simulink model "gm_tx80211a6l_interface"  (R2015b)
settings: Solver=FixedStepDiscrete  SolverMode=SingleTasking  StartTime=0.0  StopTime=46*tpf  RelTol=1e-3
PreLoadFcn:
  | [stx, stb, spi, spq, ntf, cii, cpp, css] = tx80211a_r0;
InitFcn:
  | if ~exist('srx','var')
  | [stx, stb, spi, spq, ntf, cii, cpp, css] = tx80211a_r0;
  | end
  | bitrate = 6e6; % 6 Mbits per second
  | crf = 2; % constant redundancy factor (from conv enc)
  | nepsc = 16; % #empty+pilot subcarriers
  | ncps = 16; % #cyclic prefix samples
  | ndbpf = 24; % #data bits per frame
  | ncbpf = ndbpf * crf; % #coded bits per frame
  | nscpf = ncbpf + nepsc; % #subcarriers per frame
  | nspf = nscpf + 16; % #samples per frame
  | tps = 1e-6; %tpf/nspf; % sample time
  | tpf = tps*nspf; %ndbpf/bitrate; % frame time
undefined symbols (not defined in the file): AXI4, css, Lite, ntf, stb
libraries: hdlsllib x30, simulink x13, axiinterfacelib x4, dspsigops x2
settings Model: SimulationMode=external  Creator=wchen  LastModifiedBy=bdroz
settings SolverCC: PositivePriorityOrder=on
settings DataIOCC: SaveFormat=Array  SaveOutput=off  SignalLogging=off  SaveTime=off
settings OptimizationCC: BlockReduction=off  ConditionallyExecuteInputs=off  ExpressionDepthLimit=2147483647  OptimizeModelRefInitCode=on  LifeSpan=1  MaxStackSize=64
settings DebuggingCC: AlgebraicLoopMsg=error  UnderspecifiedInitializationDetection=Classic  MergeDetectMultiDrivingBlocksExec=none  SolverPrmCheckMsg=warning  SingleTaskRateTransMsg=error  ParameterPrecisionLossMsg=none  AllowSymbolicDim=on  StateNameClashWarn=warning
settings HardwareCC: ProdBitPerPointer=32  ProdLargestAtomicInteger=Long  ProdLargestAtomicFloat=Double  ProdWordSize=32  ProdHWDeviceType=ARM Compatible->ARM Cortex  TargetBitPerPointer=64  TargetLongLongMode=on  TargetIntDivRoundTo=Zero  TargetEndianess=LittleEndian  TargetWordSize=64  TargetHWDeviceType=MATLAB Host
settings RTWCC: SystemTargetFile=ert.tlc  TemplateMakefile=ert_default_tmf  Description=Embedded Coder  GenerateReport=on  Toolchain=Xilinx Software Development Kit (SDK)  IncludeHyperlinkInReport=on  LaunchReport=on  GenerateTraceInfo=on  GenerateTraceReport=on  GenerateTraceReportSl=on  GenerateTraceReportSf=on  GenerateTraceReportEml=on
settings CodeAppCC: ForceParamTrailComments=on  IgnoreCustomStorageClasses=off  OperatorAnnotations=on  SimulinkDataObjDesc=on  SFDataObjDesc=on  MATLABFcnDesc=on  InsertBlockDesc=on  MATLABSourceComments=on
settings ERTTargetCC: ConvertIfToSwitch=on  SuppressUnreachableDefaultCases=on
settings ConfigComp: CovModelRefEnable=Off

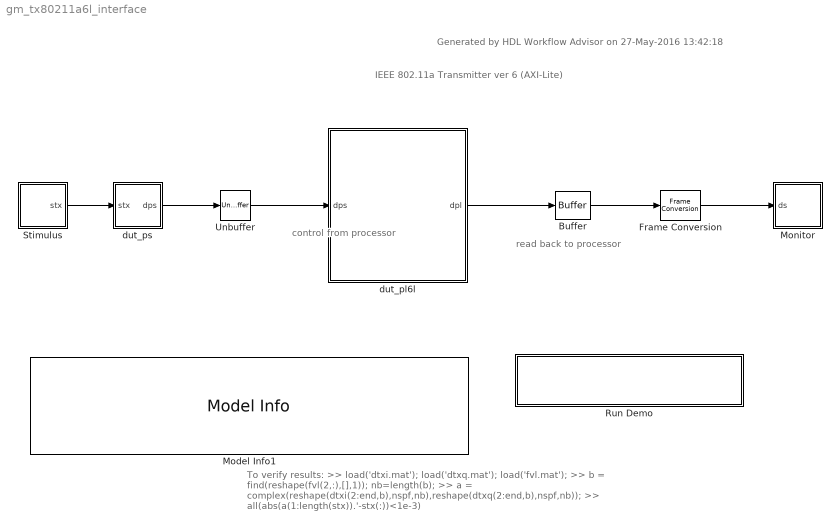
== system gm_tx80211a6l_interface ==
  note: To verify results:
      | >> load('dtxi.mat'); load('dtxq.mat'); load('fvl.mat');
      | >> b = find(reshape(fvl(2,:),[],1)); nb=length(b);
      | >> a = complex(reshape(dtxi(2:end,b),nspf,nb),reshape(dtxq(2:end,b),nspf,nb));
      | >> all(abs(a(1:length(stx)).'-stx(:))<1e-3)
  note: read back to
      | processor
  note: IEEE 802.11a Transmitter ver 6 (AXI-Lite)
  note: control from
      | processor
  note: Generated by HDL Workflow Advisor on 27-May-2016 13:42:18
  Buffer : Buffer  N=nspf  TreatMby1Signals=One channel  OutputFrames=off
  Frame Conversion : FrameConversion  InheritSamplingMode=off  OutFrame=Sample-based
  Model Info1 : simulink/Model-Wide Utilities/Model Info  Frame=on  DisplayStringWithTags=|  HorizontalTextAlignment=Left  LeftAlignmentValue=0.02  SourceBlockDiagram=gm_tx80211a6l_interface  TagMaxNumber=20
      | This example shows how to use HDL Workflow Advisor to 
      | generate a custom IP core for Zynq SoC evaluation board.
      | 
      | In MATLAB, type the following:
      |   hdladvisor('tx80211a6l/dut_pl6l')
  Monitor : Subsystem
  Run Demo : Subsystem
      settings: OpenFcn=hdladvisor([bdroot, '/led_counter'])
      mask Display: disp('Launch HDL Workflow Advisor')
  Stimulus : Subsystem
  Unbuffer : Unbuffer  SampleBasedProcessing=Same as frame based
  dut_pl6l : Subsystem  TreatAsAtomicUnit=on  mask(AXI4-Lite/AXI4 Interface){}
      mask help:
      | This is an automatically generated subsystem block.
      | This contains the AXI interface blocks that communicate with the tx80211a6l_dut_pl6l_ipcore IPCore generated from tx80211a6l/dut_pl6l subsystem.
      mask Display: disp(sprintf('Xilinx Zynq \nAXI Interface'));
  dut_ps : Subsystem
  wires:
  Frame Conversion/1 -> Monitor/1(ds)
  Unbuffer/1 -> dut_pl6l/1(dps)
  dut_ps/1(dps) -> Unbuffer/1
  Stimulus/1(stx) -> dut_ps/1(stx)
  dut_pl6l/1(dpl) -> Buffer/1
  Buffer/1 -> Frame Conversion/1

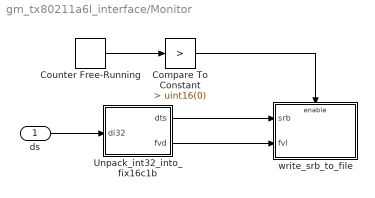
== system gm_tx80211a6l_interface/Monitor ==
  ds : Inport
  Compare To Constant : simulink/Logic and Bit Operations/Compare To Constant  relop=>  const=uint16(0)  OutDataTypeStr=boolean
  Counter Free-Running : simulink/Sources/Counter Free-Running  NumBits=16  tsamp=tpf
  Unpack_int32_into_fix16c1b : Subsystem
  write_srb_to_file : Subsystem
  wires:
  Unpack_int32_into_fix16c1b/1(dts) -> write_srb_to_file/1(srb)
  Unpack_int32_into_fix16c1b/2(fvd) -> write_srb_to_file/2(fvl)
  ds/1 -> Unpack_int32_into_fix16c1b/1(di32)
  Counter Free-Running/1 -> Compare To Constant/1
  Compare To Constant/1 -> write_srb_to_file/Enable

== system gm_tx80211a6l_interface/Run Demo ==

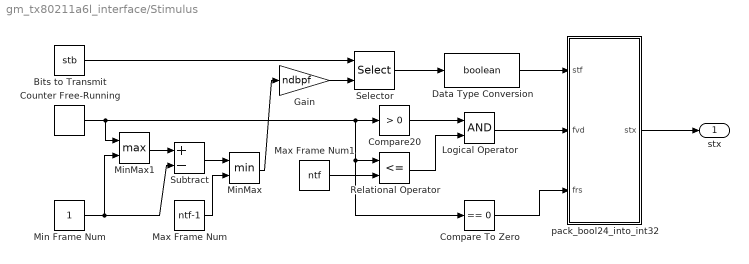
== system gm_tx80211a6l_interface/Stimulus ==
  Bits to Transmit : Constant  Value=stb  SampleTime=tpf
  Compare To Zero : simulink/Logic and Bit Operations/Compare To Zero  relop===  OutDataTypeStr=boolean
  Compare20 : simulink/Logic and Bit Operations/Compare To Zero  relop=>  OutDataTypeStr=boolean
  Counter Free-Running : simulink/Sources/Counter Free-Running  NumBits=16  tsamp=tpf
  Data Type Conversion : DataTypeConversion  OutDataTypeStr=boolean
  Gain : Gain  Gain=ndbpf  OutDataTypeStr=uint16
  Logical Operator : Logic  AllPortsSameDT=off  OutDataTypeStr=boolean
  Max Frame Num : Constant  Value=ntf-1  OutDataTypeStr=uint16  SampleTime=tpf
  Max Frame Num1 : Constant  Value=ntf  OutDataTypeStr=uint16  SampleTime=tpf
  Min Frame Num : Constant  OutDataTypeStr=uint16  SampleTime=tpf
  MinMax : MinMax  Inputs=2  OutDataTypeStr=uint16
  MinMax1 : MinMax  Function=max  Inputs=2
  Relational Operator : RelationalOperator  Operator=<=  OutDataTypeStr=boolean
  Selector : Selector  IndexMode=Zero-based  InputPortWidth=864  IndexOptions=Starting index (port)  Indices=[1 3]  OutputSizes=24
  Subtract : Sum  Inputs=+-  OutDataTypeStr=uint16
  pack_bool24_into_int32 : Subsystem
  stx : Outport
  wires:
  Max Frame Num1/1 -> Relational Operator/2
  Logical Operator/1 -> pack_bool24_into_int32/2(fvd)
  Relational Operator/1 -> Logical Operator/2
  Compare20/1 -> Logical Operator/1
  Counter Free-Running/1 -> MinMax1/1, Compare To Zero/1, Relational Operator/1, Compare20/1
  Max Frame Num/1 -> MinMax/2
  MinMax/1 -> Gain/1
  Bits to Transmit/1 -> Selector/1
  Gain/1 -> Selector/2
  Selector/1 -> Data Type Conversion/1
  Data Type Conversion/1 -> pack_bool24_into_int32/1(stf)
  pack_bool24_into_int32/1(stx) -> stx/1
  Min Frame Num/1 -> Subtract/2, MinMax1/2
  Subtract/1 -> MinMax/1
  MinMax1/1 -> Subtract/1
  Compare To Zero/1 -> pack_bool24_into_int32/3(frs)

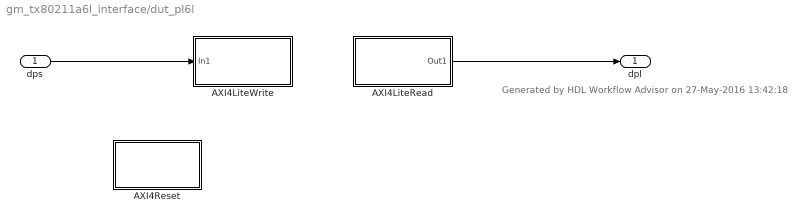
== system gm_tx80211a6l_interface/dut_pl6l ==
  note: Generated by HDL Workflow Advisor on 27-May-2016 13:42:18
  dps : Inport
  AXI4LiteRead : Subsystem  Priority=10
  AXI4LiteWrite : Subsystem  Priority=1
  AXI4Reset : Subsystem  mask(System Initialize){ShowInLibBrowser=0}
      mask prompts: ShowInLibBrowser "Simulink:masks:CustCodeMaskParam1_MP"
      settings: CopyFcn=cccopyfcn(gcb)  OpenFcn=ccopenfcn('System Initialize Function')
      mask Help: eval('feval(''rtwprivate'',''rtwhelpview'',''rtw_sys_initialize_block'')');
      mask Display: disp('System\nInitialize');
  dpl : Outport  InitialOutput=0
  wires:
  dps/1 -> AXI4LiteWrite/1(In1)
  AXI4LiteRead/1(Out1) -> dpl/1

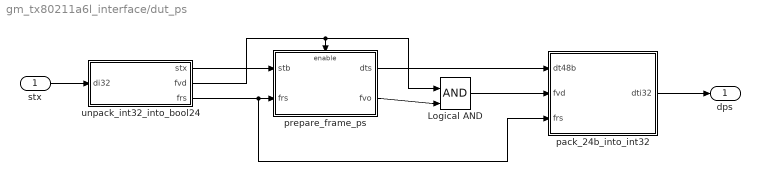
== system gm_tx80211a6l_interface/dut_ps ==
  stx : Inport
  Logical AND : Logic  IconShape=distinctive  AllPortsSameDT=off  OutDataTypeStr=boolean
  pack_24b_into_int32 : Subsystem
  prepare_frame_ps : Subsystem  TreatAsAtomicUnit=on
  unpack_int32_into_bool24 : Subsystem
  dps : Outport
  wires:
  prepare_frame_ps/2(fvo) -> Logical AND/2
  Logical AND/1 -> pack_24b_into_int32/2(fvd)
  pack_24b_into_int32/1(dti32) -> dps/1
  prepare_frame_ps/1(dts) -> pack_24b_into_int32/1(dt48b)
  unpack_int32_into_bool24/2(fvd) -> prepare_frame_ps/Enable, Logical AND/1
  unpack_int32_into_bool24/1(stx) -> prepare_frame_ps/1(stb)
  unpack_int32_into_bool24/3(frs) -> prepare_frame_ps/2(frs), pack_24b_into_int32/3(frs)
  stx/1 -> unpack_int32_into_bool24/1(di32)

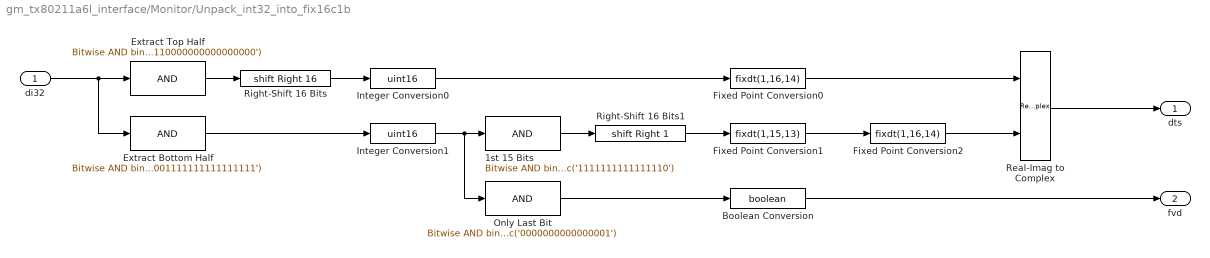
== system gm_tx80211a6l_interface/Monitor/Unpack_int32_into_fix16c1b ==
  di32 : Inport
  1st 15 Bits : simulink/Logic and Bit Operations/Bitwise Operator  logicop=AND  UseBitMask=on  BitMask=bin2dec('1111111111111110')  BitMaskRealWorld=Stored Integer
  Boolean Conversion : DataTypeConversion  OutDataTypeStr=boolean  ConvertRealWorld=Stored Integer (SI)
  Extract Bottom Half : simulink/Logic and Bit Operations/Bitwise Operator  logicop=AND  UseBitMask=on  BitMask=bin2dec('00000000000000001111111111111111')  BitMaskRealWorld=Stored Integer
  Extract Top Half : simulink/Logic and Bit Operations/Bitwise Operator  logicop=AND  UseBitMask=on  BitMask=bin2dec('11111111111111110000000000000000')  BitMaskRealWorld=Stored Integer
  Fixed Point Conversion0 : DataTypeConversion  OutDataTypeStr=fixdt(1,16,14)  ConvertRealWorld=Stored Integer (SI)
      settings: AttributesFormatString=%<OutDataTypeStr>
  Fixed Point Conversion1 : DataTypeConversion  OutDataTypeStr=fixdt(1,15,13)  ConvertRealWorld=Stored Integer (SI)
      settings: AttributesFormatString=%<OutDataTypeStr>
  Fixed Point Conversion2 : DataTypeConversion  OutDataTypeStr=fixdt(1,16,14)
      settings: AttributesFormatString=%<OutDataTypeStr>
  Integer Conversion0 : DataTypeConversion  OutDataTypeStr=uint16  ConvertRealWorld=Stored Integer (SI)
  Integer Conversion1 : DataTypeConversion  OutDataTypeStr=uint16  ConvertRealWorld=Stored Integer (SI)
  Only Last Bit : simulink/Logic and Bit Operations/Bitwise Operator  logicop=AND  UseBitMask=on  BitMask=bin2dec('0000000000000001')  BitMaskRealWorld=Stored Integer
  Real-Imag to Complex : RealImagToComplex
  Right-Shift 16 Bits : ArithShift  BitShiftNumber=16  BitShiftDirection=Right  DiagnosticForOORShift=Error
  Right-Shift 16 Bits1 : ArithShift  BitShiftNumber=1  BitShiftDirection=Right  DiagnosticForOORShift=Error
  dts : Outport
  fvd : Outport  Port=2
  wires:
  Right-Shift 16 Bits1/1 -> Fixed Point Conversion1/1
  Fixed Point Conversion1/1 -> Fixed Point Conversion2/1
  Integer Conversion0/1 -> Fixed Point Conversion0/1
  Integer Conversion1/1 -> Only Last Bit/1, 1st 15 Bits/1
  Extract Top Half/1 -> Right-Shift 16 Bits/1
  Right-Shift 16 Bits/1 -> Integer Conversion0/1
  1st 15 Bits/1 -> Right-Shift 16 Bits1/1
  di32/1 -> Extract Top Half/1, Extract Bottom Half/1
  Extract Bottom Half/1 -> Integer Conversion1/1
  Fixed Point Conversion2/1 -> Real-Imag to Complex/2
  Fixed Point Conversion0/1 -> Real-Imag to Complex/1
  Boolean Conversion/1 -> fvd/1
  Only Last Bit/1 -> Boolean Conversion/1
  Real-Imag to Complex/1 -> dts/1

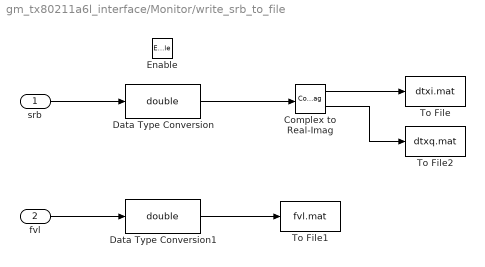
== system gm_tx80211a6l_interface/Monitor/write_srb_to_file ==
  srb : Inport
  fvl : Inport  Port=2
  Enable : EnablePort
  Complex to Real-Imag : ComplexToRealImag
  Data Type Conversion : DataTypeConversion  OutDataTypeStr=double
  Data Type Conversion1 : DataTypeConversion  OutDataTypeStr=double
  To File : ToFile  Filename=dtxi.mat  MatrixName=dtxi  SampleTime=tpf
  To File1 : ToFile  Filename=fvl.mat  MatrixName=fvl  SampleTime=tpf
  To File2 : ToFile  Filename=dtxq.mat  MatrixName=dtxq  SampleTime=tpf
  wires:
  Complex to Real-Imag/2 -> To File2/1
  Complex to Real-Imag/1 -> To File/1
  Data Type Conversion/1 -> Complex to Real-Imag/1
  srb/1 -> Data Type Conversion/1
  Data Type Conversion1/1 -> To File1/1
  fvl/1 -> Data Type Conversion1/1

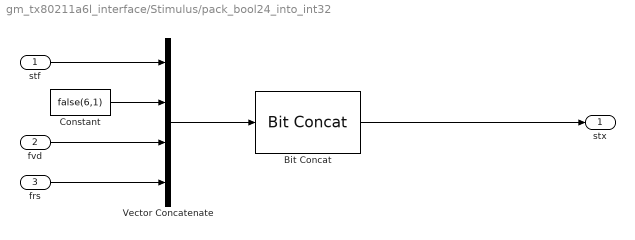
== system gm_tx80211a6l_interface/Stimulus/pack_bool24_into_int32 ==
  stf : Inport
  fvd : Inport  Port=2
  frs : Inport  Port=3
  Bit Concat : hdlsllib/HDL Operations/Bit Concat  numInputs=1
  Constant : Constant  Value=false(6,1)  OutDataTypeStr=boolean  SampleTime=tpf
  Vector Concatenate : Concatenate  NumInputs=4
  stx : Outport
  wires:
  Bit Concat/1 -> stx/1
  Constant/1 -> Vector Concatenate/2
  frs/1 -> Vector Concatenate/4
  fvd/1 -> Vector Concatenate/3
  stf/1 -> Vector Concatenate/1
  Vector Concatenate/1 -> Bit Concat/1

== system gm_tx80211a6l_interface/dut_pl6l/AXI4LiteRead ==
  AXI4Lite_Read_dpl : axiinterfacelib/AXI4-Interface Read  Priority=2  AXIInterfaceType=AXI4-Lite  DeviceName=/dev/mwipcore  RegisterOffset=hex2dec('104')  DataLength=4096  DataType=uint32  SampleTime=-1  blockPlatform=ZYNQ  SimulateUsing=Interpreted Execution
  AXI4Lite_Read_dpl_DTC : DataTypeConversion  OutDataTypeStr=fixdt('uint32')  ConvertRealWorld=Stored Integer (SI)
  AXI4_Handshake : Subsystem  Priority=1  mask(AXI4-Lite/AXI4 Handshake){blockPlatform=ZYNQ}
      mask prompts: blockPlatform "Mask Parameter 1:"
      mask help:
      | This is an automatically generated block.
      | It synchronizes the data between ARM and FPGA on AXI4-Lite/AXI4 interface.
      |
      | This block writes the FPGA Strobe signal to indicate that the data from ARM on AXI4-Lite/AXI4 interface is valid.
      |
      | It waits until the FPGA Ready signal is 1 (logic-HIGH), which shows that data from FPGA on AXI4-Lite/AXI4 interface is valid.
      mask Display:
      | color('blue');
      | text(0.67, 0.87, 'ZYNQ', 'horizontalAlignment', 'left');
  Out1 : Outport
  wires:
  AXI4Lite_Read_dpl_DTC/1 -> Out1/1
  AXI4Lite_Read_dpl/1 -> AXI4Lite_Read_dpl_DTC/1

== system gm_tx80211a6l_interface/dut_pl6l/AXI4LiteWrite ==
  In1 : Inport
  AXI4Lite_Write_dps : axiinterfacelib/AXI4-Interface Write  Priority=1  AXIInterfaceType=AXI4-Lite  DeviceName=/dev/mwipcore  RegisterOffset=hex2dec('100')  blockPlatform=ZYNQ  SimulateUsing=Interpreted execution
  AXI4Lite_Write_dps_DTC : DataTypeConversion  OutDataTypeStr=uint32  ConvertRealWorld=Stored Integer (SI)
  wires:
  AXI4Lite_Write_dps_DTC/1 -> AXI4Lite_Write_dps/1
  In1/1 -> AXI4Lite_Write_dps_DTC/1

== system gm_tx80211a6l_interface/dut_pl6l/AXI4Reset ==

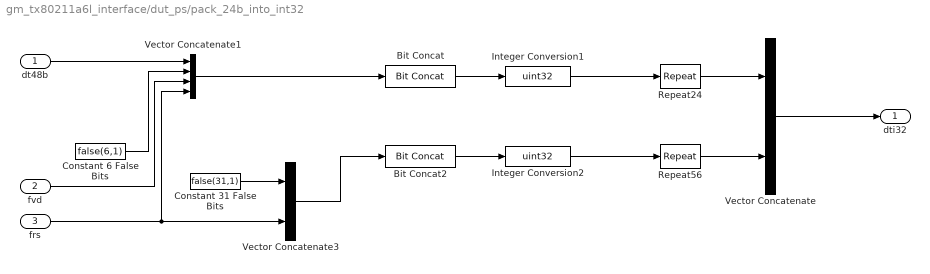
== system gm_tx80211a6l_interface/dut_ps/pack_24b_into_int32 ==
  dt48b : Inport
  fvd : Inport  Port=2
  frs : Inport  Port=3
  Bit Concat : hdlsllib/HDL Operations/Bit Concat  numInputs=1
  Bit Concat2 : hdlsllib/HDL Operations/Bit Concat  numInputs=1
  Constant 31 False Bits : Constant  Value=false(31,1)  OutDataTypeStr=boolean  SampleTime=tpf
  Constant 6 False Bits : Constant  Value=false(6,1)  OutDataTypeStr=boolean  SampleTime=tpf
  Integer Conversion1 : DataTypeConversion  OutDataTypeStr=uint32  ConvertRealWorld=Stored Integer (SI)
  Integer Conversion2 : DataTypeConversion  OutDataTypeStr=uint32  ConvertRealWorld=Stored Integer (SI)
  Repeat24 : dspsigops/Repeat  N=24  InputProcessing=Columns as channels (frame based)  RateOptions=Enforce single-rate processing  ic=0  mode=Unused parameter value
  Repeat56 : dspsigops/Repeat  N=56  InputProcessing=Columns as channels (frame based)  RateOptions=Enforce single-rate processing  ic=0  mode=Unused parameter value
  Vector Concatenate : Concatenate
  Vector Concatenate1 : Concatenate  NumInputs=4
  Vector Concatenate3 : Concatenate
  dti32 : Outport
  wires:
  Repeat24/1 -> Vector Concatenate/1
  Integer Conversion1/1 -> Repeat24/1
  Repeat56/1 -> Vector Concatenate/2
  Integer Conversion2/1 -> Repeat56/1
  Bit Concat2/1 -> Integer Conversion2/1
  Vector Concatenate3/1 -> Bit Concat2/1
  Constant 31 False Bits/1 -> Vector Concatenate3/1
  Constant 6 False Bits/1 -> Vector Concatenate1/2
  Vector Concatenate1/1 -> Bit Concat/1
  frs/1 -> Vector Concatenate3/2, Vector Concatenate1/4
  fvd/1 -> Vector Concatenate1/3
  dt48b/1 -> Vector Concatenate1/1
  Bit Concat/1 -> Integer Conversion1/1
  Vector Concatenate/1 -> dti32/1

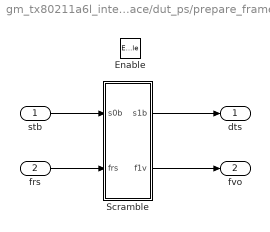
== system gm_tx80211a6l_interface/dut_ps/prepare_frame_ps ==
  stb : Inport
  frs : Inport  Port=2
  Enable : EnablePort
  Scramble : Subsystem  TreatAsAtomicUnit=on
  dts : Outport
  fvo : Outport  Port=2  InitialOutput=0
  wires:
  Scramble/1(s1b) -> dts/1
  Scramble/2(f1v) -> fvo/1
  frs/1 -> Scramble/2(frs)
  stb/1 -> Scramble/1(s0b)

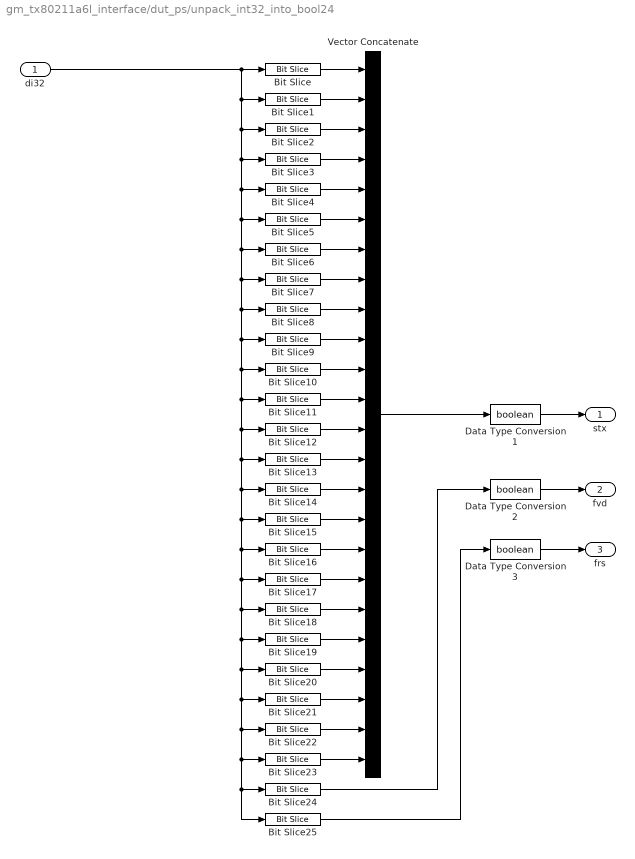
== system gm_tx80211a6l_interface/dut_ps/unpack_int32_into_bool24 ==
  di32 : Inport
  Bit Slice : hdlsllib/HDL Operations/Bit Slice  lidx=31  ridx=31
      settings: AttributesFormatString=%<lidx>
  Bit Slice1 : hdlsllib/HDL Operations/Bit Slice  lidx=30  ridx=30
      settings: AttributesFormatString=%<lidx>
  Bit Slice10 : hdlsllib/HDL Operations/Bit Slice  lidx=21  ridx=21
      settings: AttributesFormatString=%<lidx>
  Bit Slice11 : hdlsllib/HDL Operations/Bit Slice  lidx=20  ridx=20
      settings: AttributesFormatString=%<lidx>
  Bit Slice12 : hdlsllib/HDL Operations/Bit Slice  lidx=19  ridx=19
      settings: AttributesFormatString=%<lidx>
  Bit Slice13 : hdlsllib/HDL Operations/Bit Slice  lidx=18  ridx=18
      settings: AttributesFormatString=%<lidx>
  Bit Slice14 : hdlsllib/HDL Operations/Bit Slice  lidx=17  ridx=17
      settings: AttributesFormatString=%<lidx>
  Bit Slice15 : hdlsllib/HDL Operations/Bit Slice  lidx=16  ridx=16
      settings: AttributesFormatString=%<lidx>
  Bit Slice16 : hdlsllib/HDL Operations/Bit Slice  lidx=15  ridx=15
      settings: AttributesFormatString=%<lidx>
  Bit Slice17 : hdlsllib/HDL Operations/Bit Slice  lidx=14  ridx=14
      settings: AttributesFormatString=%<lidx>
  Bit Slice18 : hdlsllib/HDL Operations/Bit Slice  lidx=13  ridx=13
      settings: AttributesFormatString=%<lidx>
  Bit Slice19 : hdlsllib/HDL Operations/Bit Slice  lidx=12  ridx=12
      settings: AttributesFormatString=%<lidx>
  Bit Slice2 : hdlsllib/HDL Operations/Bit Slice  lidx=29  ridx=29
      settings: AttributesFormatString=%<lidx>
  Bit Slice20 : hdlsllib/HDL Operations/Bit Slice  lidx=11  ridx=11
      settings: AttributesFormatString=%<lidx>
  Bit Slice21 : hdlsllib/HDL Operations/Bit Slice  lidx=10  ridx=10
      settings: AttributesFormatString=%<lidx>
  Bit Slice22 : hdlsllib/HDL Operations/Bit Slice  lidx=9  ridx=9
      settings: AttributesFormatString=%<lidx>
  Bit Slice23 : hdlsllib/HDL Operations/Bit Slice  lidx=8  ridx=8
      settings: AttributesFormatString=%<lidx>
  Bit Slice24 : hdlsllib/HDL Operations/Bit Slice  lidx=1  ridx=1
      settings: AttributesFormatString=%<lidx>
  Bit Slice25 : hdlsllib/HDL Operations/Bit Slice  lidx=0  ridx=0
      settings: AttributesFormatString=%<lidx>
  Bit Slice3 : hdlsllib/HDL Operations/Bit Slice  lidx=28  ridx=28
      settings: AttributesFormatString=%<lidx>
  Bit Slice4 : hdlsllib/HDL Operations/Bit Slice  lidx=27  ridx=27
      settings: AttributesFormatString=%<lidx>
  Bit Slice5 : hdlsllib/HDL Operations/Bit Slice  lidx=26  ridx=26
      settings: AttributesFormatString=%<lidx>
  Bit Slice6 : hdlsllib/HDL Operations/Bit Slice  lidx=25  ridx=25
      settings: AttributesFormatString=%<lidx>
  Bit Slice7 : hdlsllib/HDL Operations/Bit Slice  lidx=24  ridx=24
      settings: AttributesFormatString=%<lidx>
  Bit Slice8 : hdlsllib/HDL Operations/Bit Slice  lidx=23  ridx=23
      settings: AttributesFormatString=%<lidx>
  Bit Slice9 : hdlsllib/HDL Operations/Bit Slice  lidx=22  ridx=22
      settings: AttributesFormatString=%<lidx>
  Data Type Conversion1 : DataTypeConversion  OutDataTypeStr=boolean
  Data Type Conversion2 : DataTypeConversion  OutDataTypeStr=boolean
  Data Type Conversion3 : DataTypeConversion  OutDataTypeStr=boolean
  Vector Concatenate : Concatenate  NumInputs=24
  stx : Outport
  fvd : Outport  Port=2
  frs : Outport  Port=3
  wires:
  Data Type Conversion3/1 -> frs/1
  Data Type Conversion2/1 -> fvd/1
  Data Type Conversion1/1 -> stx/1
  Bit Slice/1 -> Vector Concatenate/1
  Bit Slice1/1 -> Vector Concatenate/2
  Bit Slice2/1 -> Vector Concatenate/3
  Bit Slice3/1 -> Vector Concatenate/4
  Bit Slice4/1 -> Vector Concatenate/5
  Bit Slice5/1 -> Vector Concatenate/6
  Bit Slice6/1 -> Vector Concatenate/7
  Bit Slice7/1 -> Vector Concatenate/8
  Bit Slice8/1 -> Vector Concatenate/9
  Bit Slice9/1 -> Vector Concatenate/10
  Bit Slice10/1 -> Vector Concatenate/11
  Bit Slice11/1 -> Vector Concatenate/12
  Bit Slice12/1 -> Vector Concatenate/13
  Bit Slice13/1 -> Vector Concatenate/14
  Bit Slice14/1 -> Vector Concatenate/15
  Bit Slice15/1 -> Vector Concatenate/16
  Bit Slice16/1 -> Vector Concatenate/17
  Bit Slice17/1 -> Vector Concatenate/18
  Bit Slice18/1 -> Vector Concatenate/19
  Bit Slice19/1 -> Vector Concatenate/20
  Bit Slice20/1 -> Vector Concatenate/21
  Bit Slice21/1 -> Vector Concatenate/22
  Bit Slice22/1 -> Vector Concatenate/23
  Bit Slice23/1 -> Vector Concatenate/24
  di32/1 -> Bit Slice/1, Bit Slice6/1, Bit Slice10/1, Bit Slice14/1, Bit Slice16/1, Bit Slice22/1, Bit Slice23/1, Bit Slice24/1, Bit Slice25/1, Bit Slice21/1, Bit Slice20/1, Bit Slice19/1, Bit Slice18/1, Bit Slice17/1, Bit Slice15/1, Bit Slice13/1, Bit Slice12/1, Bit Slice11/1, Bit Slice9/1, Bit Slice8/1, Bit Slice7/1, Bit Slice5/1, Bit Slice4/1, Bit Slice3/1, Bit Slice2/1, Bit Slice1/1
  Bit Slice24/1 -> Data Type Conversion2/1
  Bit Slice25/1 -> Data Type Conversion3/1
  Vector Concatenate/1 -> Data Type Conversion1/1

== system gm_tx80211a6l_interface/dut_pl6l/AXI4LiteRead/AXI4_Handshake ==
  AXI4_Write_FPGA_STROBE : axiinterfacelib/AXI4-Interface Write  Priority=1  AXIInterfaceType=AXI4-Lite  DeviceName=/dev/mwipcore  RegisterOffset=hex2dec('8')  blockPlatform=ZYNQ  SimulateUsing=Interpreted execution
  Constant : Constant  OutDataTypeStr=uint32
  WhileIteratorSubsystem : Subsystem  Priority=10  TreatAsAtomicUnit=on
  wires:
  Constant/1 -> AXI4_Write_FPGA_STROBE/1

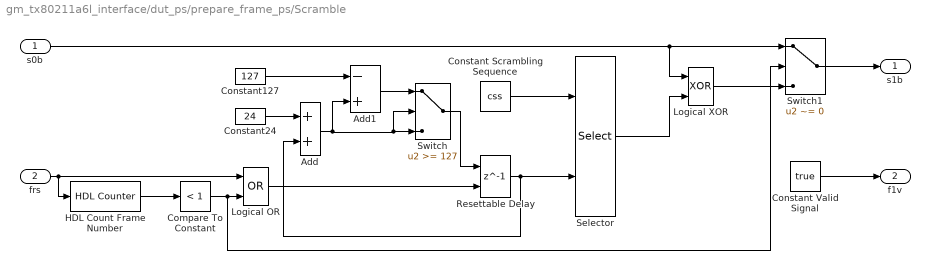
== system gm_tx80211a6l_interface/dut_ps/prepare_frame_ps/Scramble ==
  s0b : Inport
  frs : Inport  Port=2
  Add : Sum  AccumDataTypeStr=int16  OutDataTypeStr=int16  SaturateOnIntegerOverflow=on
  Add1 : Sum  Inputs=-+  AccumDataTypeStr=int16  OutDataTypeStr=int16  SaturateOnIntegerOverflow=on  LockScale=on
  Compare To Constant : simulink/Logic and Bit Operations/Compare To Constant  relop=<  const=1  OutDataTypeStr=boolean
  Constant Scrambling Sequence : Constant  Value=css  OutDataTypeStr=boolean  SampleTime=tpf
  Constant Valid Signal : Constant  Value=true  OutDataTypeStr=boolean  SampleTime=tpf
  Constant127 : Constant  Value=127  OutDataTypeStr=int16  SampleTime=tpf
  Constant24 : Constant  Value=24  OutDataTypeStr=int16  SampleTime=tpf
  HDL Count Frame Number : hdlsllib/HDL Operations/HDL Counter  CountType=Free running  CountInit=0  CountStep=1  CountMax=25  CountFromType=Initial value  CountFrom=0  CountResetPort=on  CountLoadPort=off  CountEnbPort=off  CountDirPort=off  CountDataType=Unsigned  CountWordLen=16  CountFracLen=0  CountSampTime=1
  Logical OR : Logic  Operator=OR  IconShape=distinctive  AllPortsSameDT=off  OutDataTypeStr=boolean
  Logical XOR : Logic  Operator=XOR  IconShape=distinctive  AllPortsSameDT=off  OutDataTypeStr=boolean
  Resettable Delay : Delay  DelayLength=1  InitialCondition=int16(0)  ExternalReset=Level  SampleTime=tpf
      settings: InputPortMap=u0,r5
  Selector : Selector  IndexMode=Zero-based  InputPortWidth=254  IndexOptions=Starting index (port)  Indices=[1 3]  OutputSizes=24
  Switch : Switch  Threshold=127
  Switch1 : Switch  Criteria=u2 ~= 0
  s1b : Outport
  f1v : Outport  Port=2
  wires:
  Switch1/1 -> s1b/1
  Logical XOR/1 -> Switch1/3
  Logical OR/1 -> Resettable Delay/2
  Constant127/1 -> Add1/1
  Add1/1 -> Switch/1
  Add/1 -> Switch/3, Switch/2, Add1/2
  Switch/1 -> Resettable Delay/1
  Constant24/1 -> Add/1
  Constant Valid Signal/1 -> f1v/1
  Selector/1 -> Logical XOR/2
  Constant Scrambling Sequence/1 -> Selector/1
  Resettable Delay/1 -> Selector/2, Add/2
  Compare To Constant/1 -> Logical OR/2, Switch1/2
  HDL Count Frame Number/1 -> Compare To Constant/1
  frs/1 -> Logical OR/1, HDL Count Frame Number/1
  s0b/1 -> Logical XOR/1, Switch1/1

== system gm_tx80211a6l_interface/dut_pl6l/AXI4LiteRead/AXI4_Handshake/WhileIteratorSubsystem ==
  AXI4_Read_FPGA_READY : axiinterfacelib/AXI4-Interface Read  Priority=1  AXIInterfaceType=AXI4-Lite  DeviceName=/dev/mwipcore  RegisterOffset=hex2dec('C')  DataLength=4096  DataType=uint32  SampleTime=-1  blockPlatform=ZYNQ  SimulateUsing=Interpreted Execution
  Compare_To_Zero : simulink/Logic and Bit Operations/Compare To Zero  relop===  OutDataTypeStr=boolean
  Constant_SimMode : Constant  OutDataTypeStr=uint32
  EnvController : simulink/Signal Routing/Environment Controller
  While Iterator : WhileIterator  MaxIters=-1  WhileBlockType=do-while  ResetStates=reset
  wires:
  Constant_SimMode/1 -> EnvController/1
  AXI4_Read_FPGA_READY/1 -> EnvController/2
  EnvController/1 -> Compare_To_Zero/1
  Compare_To_Zero/1 -> While Iterator/1
